simulink model "Ejercicio9"  (R2012b)
settings: Solver=ode45  StartTime=0.0  StopTime=20  RelTol=1e-3
values from neighbouring files (symbols this model uses):
  a = [-1 -3 -1; -2 -4 -1;2 -2 -3]    [ejercicio9.m]
  b = [3; 2 ;2]    [ejercicio9.m]
  c = [1 0 1]    [ejercicio9.m]
  h = h'    [ejercicio9.m]
  k = place(a,b,[pd' -22])    [ejercicio9.m]
settings Model: Creator=mario  LastModifiedBy=carlos_mar.paredes
settings DataIOCC: SignalLoggingSaveFormat=ModelDataLogs
settings OptimizationCC: ExpressionDepthLimit=128
settings DebuggingCC: MultiTaskDSMMsg=warning  MultiTaskCondExecSysMsg=none  StrictBusMsg=None
settings RTWCC: IncludeERTFirstTime=on
settings CodeAppCC: CustomSymbolStrType=$N$R$M_T  InternalIdentifier=Shortened

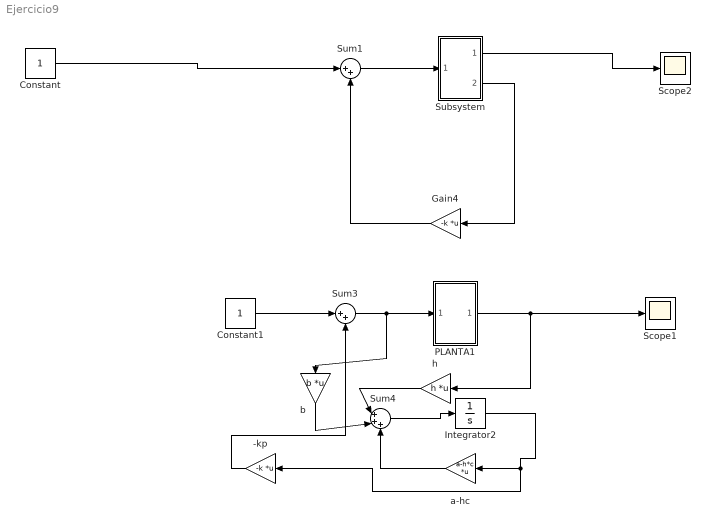
== system Ejercicio9 ==
  -kp : Gain  Gain=-k  Multiplication=Matrix(K*u) (u vector)
  Constant : Constant
  Constant1 : Constant
  Gain4 : Gain  Gain=-k  Multiplication=Matrix(K*u) (u vector)
  Integrator2 : Integrator
  PLANTA1 : Subsystem
  Scope1 : Scope
  Scope2 : Scope
  Subsystem : Subsystem
  Sum1 : Sum  Inputs=|++
  Sum3 : Sum  Inputs=|++
  Sum4 : Sum  Inputs=|+++
  a-hc : Gain  Gain=a-h*c  Multiplication=Matrix(K*u) (u vector)
  b : Gain  Gain=b  Multiplication=Matrix(K*u) (u vector)
  h : Gain  Gain=h  Multiplication=Matrix(K*u) (u vector)
  wires:
  Gain4/1 -> Sum1/2
  Constant/1 -> Sum1/1
  Subsystem/1(Out1) -> Scope2/1
  Sum1/1 -> Subsystem/1(In1)
  Subsystem/2(Out2) -> Gain4/1
  PLANTA1/1(Out1) -> h/1, Scope1/1
  Sum3/1 -> b/1, PLANTA1/1(In1)
  h/1 -> Sum4/1
  b/1 -> Sum4/2
  Sum4/1 -> Integrator2/1
  Integrator2/1 -> -kp/1, a-hc/1
  a-hc/1 -> Sum4/3
  -kp/1 -> Sum3/2
  Constant1/1 -> Sum3/1

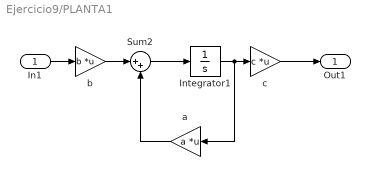
== system Ejercicio9/PLANTA1 ==
  In1 : Inport
  Integrator1 : Integrator
  Sum2 : Sum  Inputs=|++
  a : Gain  Gain=a  Multiplication=Matrix(K*u) (u vector)
  b : Gain  Gain=b  Multiplication=Matrix(K*u) (u vector)
  c : Gain  Gain=c  Multiplication=Matrix(K*u) (u vector)
  Out1 : Outport
  wires:
  Sum2/1 -> Integrator1/1
  c/1 -> Out1/1
  a/1 -> Sum2/2
  b/1 -> Sum2/1
  In1/1 -> b/1
  Integrator1/1 -> c/1, a/1

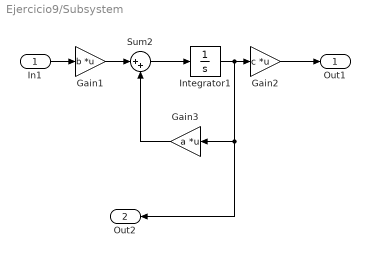
== system Ejercicio9/Subsystem ==
  In1 : Inport
  Gain1 : Gain  Gain=b  Multiplication=Matrix(K*u) (u vector)
  Gain2 : Gain  Gain=c  Multiplication=Matrix(K*u) (u vector)
  Gain3 : Gain  Gain=a  Multiplication=Matrix(K*u) (u vector)
  Integrator1 : Integrator
  Sum2 : Sum  Inputs=|++
  Out1 : Outport
  Out2 : Outport  Port=2
  wires:
  Integrator1/1 -> Out2/1, Gain3/1, Gain2/1
  In1/1 -> Gain1/1
  Gain1/1 -> Sum2/1
  Gain3/1 -> Sum2/2
  Gain2/1 -> Out1/1
  Sum2/1 -> Integrator1/1
